simulink model "model_mavic"  (R2020b)
settings: Solver=VariableStepAuto  StartTime=0.0  StopTime=10.0  RelTol=1e-3
settings Model: Creator=boringtao  LastModifiedBy=boringtao

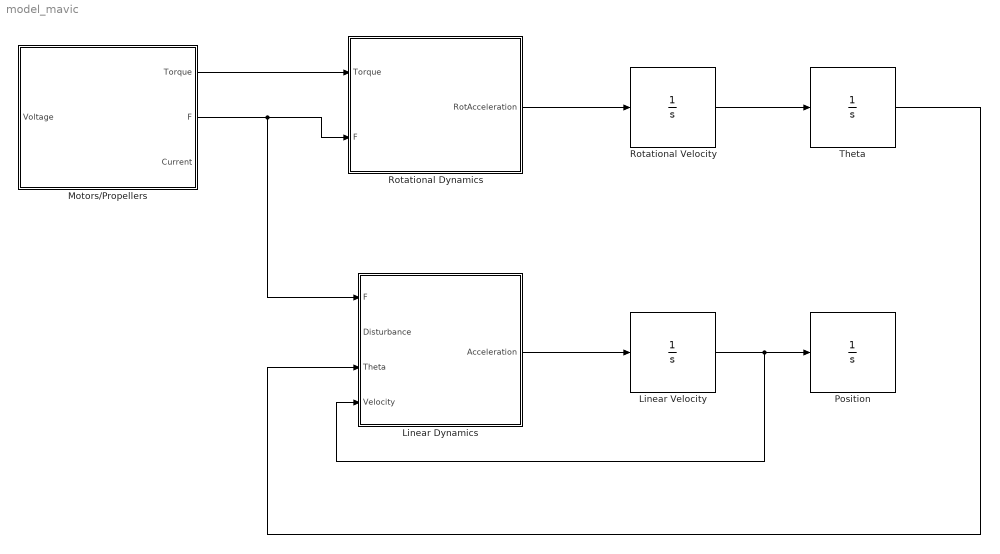
== system model_mavic ==
  Linear Dynamics : MATLAB Function  TreatAsAtomicUnit=on
  Linear Velocity : Integrator
  Motors/Propellers : MATLAB Function  TreatAsAtomicUnit=on
  Position : Integrator
  Rotational Dynamics : MATLAB Function  TreatAsAtomicUnit=on
  Rotational Velocity : Integrator
  Theta : Integrator
  wires:
  Motors/Propellers/1(Torque) -> Rotational Dynamics/1(Torque)
  Motors/Propellers/2(F) -> Rotational Dynamics/2(F), Linear Dynamics/1(F)
  Rotational Dynamics/1(RotAcceleration) -> Rotational Velocity/1
  Rotational Velocity/1 -> Theta/1
  Theta/1 -> Linear Dynamics/3(Theta)
  Linear Dynamics/1(Acceleration) -> Linear Velocity/1
  Linear Velocity/1 -> Linear Dynamics/4(Velocity), Position/1

== matlab function model_mavic/Rotational Dynamics ==
  data: Torque input; RotAcceleration output; F input
function RotAcceleration = fcn(Torque, F)
Moment = [0 0 0];
RotAcceleration = [0 0 0];
I = [0.003 0.003 0.007];

Moment(1) = (F(3) + F(4))*0.237/2 - (F(1) + F(2))*0.237/2
Moment(2) = (F(3) + F(2))*0.237/2 - (F(1) + F(4))*0.237/2
Moment(3) = Torque(4) - Torque(1) + Torque(2) - Torque(4)

for i = 1:3
    RotAcceleration(i) = Moment(i)/I(i);
end

== matlab function model_mavic/Motors//Propellers ==
  data: Voltage input; Torque output; F output; Current output
function [Torque, F, Current] = fcn(Voltage)
RPM = [0 0 0 0]
Torque = [0 0 0 0]
Current = [0 0 0 0]
F = [0 0 0 0]

for i=1:4
    RPM(i) = -2.6932*Voltage(i)^3 + 1400*Voltage(i);
    Ct = 2*10^ - 15*RPM(i)^3 - 4*10^ - 11*RPM(i)^2 + 3*10^ - 7*RPM(i) + 0.1013;
    F(i) = Ct*1.225*(RPM(i)/60)^2*0.2^4;
    Torque(i) = 4*10^ -14*RPM(i)^3 + 8*10^ -12*RPM(i)^2 + 3*10^ -6*RPM(i);
    Current(i) = 1400*Torque(i);
end

== matlab function model_mavic/Linear Dynamics ==
  data: F input; Acceleration output; Disturbance input; Theta input; Velocity input
function Acceleration = fcn(F, Disturbance, Theta, Velocity)
m = 0.743;
g = 9.81;
A = [0.0197, 0.0197, 0.0512];
rho = 1.225;
Cd = 1;

Acceleration = [0 0 0];
Force = [0 0 0];
Fprop = [0 0 0];

Fprop(1) = sin(Theta(2))*cos(Theta(1))*(F(1)+F(2)+F(3)+F(4));
Fprop(2) = sin(Theta(1))*cos(Theta(2))*(F(1)+F(2)+F(3)+F(4));
Fprop(3) = cos(Theta(2))*cos(Theta(1))*(F(1)+F(2)+F(3)+F(4));

ThetaXY = atan2(Fprop(1), Fprop(2));
XY2D = sqrt(Fprop(1)^2 + Fprop(2)^2);

if Fprop(3)>=0
    Fprop(1) = XY2D*sin(ThetaXY + Theta(3));
    Fprop(2) = XY2D*cos(ThetaXY + Theta(3));
else
    Fprop(1) = XY2D*sin(-ThetaXY + Theta(3));
    Fprop(2) = XY2D*cos(-ThetaXY + Theta(3));
end

if Velocity(1)<0
    Force(1)=Fprop(1)-Disturbance(1)+0.5*rho*Velocity(1)^2*A(1)*Cd;
else
    Force(1)=Fprop(1)-Disturbance(1)-0.5*rho*Velocity(1)^2*A(1)*Cd;
end

if Velocity(2)<0
    Force(2)=Fprop(2)-Disturbance(2)+0.5*rho*Velocity(2)^2*A(2)*Cd;
else
    Force(2)=Fprop(2)-Disturbance(2)-0.5*rho*Velocity(2)^2*A(2)*Cd;
end

if Velocity(3)<0
    Force(3)=Fprop(3)-Disturbance(3)+0.5*rho*Velocity(3)^2*A(3)*Cd-m*g;
else
    Force(3)=Fprop(3)-Disturbance(3)-0.5*rho*Velocity(3)^2*A(3)*Cd-m*g;
end

for i=1:3
    Acceleration(i)=Force(i)/m;
end
